simulink model "AccurateModelToBeChecked"  (R2024b)
settings: Solver=VariableStepAuto  StartTime=0.0  StopTime=10.0  RelTol=1e-3
settings Model: Creator=federico  LastModifiedBy=federico

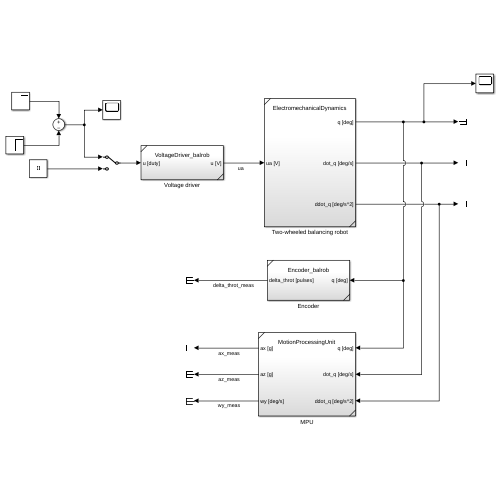
[thumbnail: Simulink's stored preview of the top-level diagram]
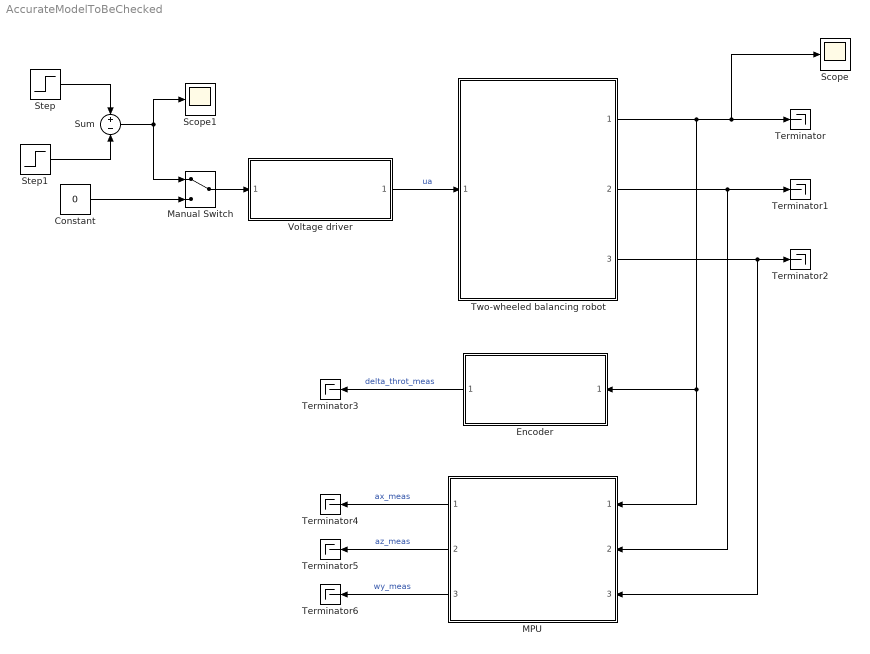
== system AccurateModelToBeChecked ==
  Constant : Constant  Value=0
  Encoder : Subsystem  ReferencedSubsystem=Encoder_balrob
  MPU : Subsystem  ReferencedSubsystem=MotionProcessingUnit
  Manual Switch : ManualSwitch
  Scope : Scope
  Scope1 : Scope
  Step : Step  After=5  SampleTime=0
  Step1 : Step  Time=1.1  After=5  SampleTime=0
  Sum : Sum  Inputs=+|-
  Terminator{,1..6} (7 alike) : Terminator
  Two-wheeled balancing robot : Subsystem  ReferencedSubsystem=ElectromechanicalDynamics
  Voltage driver : Subsystem  ReferencedSubsystem=VoltageDriver_balrob
  wires:
  Encoder/1 -> Terminator3/1  "delta_throt_meas"
  Manual Switch/1 -> Voltage driver/1
  Two-wheeled balancing robot/3 -> MPU/3, Terminator2/1
  Two-wheeled balancing robot/1 -> MPU/1, Encoder/1, Terminator/1, Scope/1
  MPU/2 -> Terminator5/1  "az_meas"
  MPU/3 -> Terminator6/1  "wy_meas"
  Voltage driver/1 -> Two-wheeled balancing robot/1  "ua"
  Constant/1 -> Manual Switch/2
  Two-wheeled balancing robot/2 -> Terminator1/1, MPU/2
  MPU/1 -> Terminator4/1  "ax_meas"
  Step/1 -> Sum/1
  Step1/1 -> Sum/2
  Sum/1 -> Scope1/1, Manual Switch/1
